simulink model "different_estimation_methods"  (R2023a)
settings: Solver=FixedStepAuto  StartTime=start_time  StopTime=stop_time  FixedStep=sample_time  RelTol=1e-3
values from neighbouring files (symbols this model uses):
  a = -0.8    [example12.m]    (also in example14.m; example15.m; example16.m)
  b = 0.5    [example12.m]    (also in example14.m; example15.m; example16.m)
  c = -0.5    [example12.m]    (also in example14.m = 0; example15.m = 0; example16.m = 0)
  e_mean = 0    [example15.m]    (also in example16.m)
  e_seed = 2    [example15.m]    (also in example16.m)
  e_var = e_std^2    (= 0.25)    [example15.m]    (also in example16.m)
  lambda = Lambda(i)    [example15.m]    (also in example16.m = 0.2)
  n_a = 1    [example15.m]    (also in example16.m)
  n_b = 1    [example15.m]    (also in example16.m)
  n_c = 0    [example15.m]    (also in example16.m = 1)
  P0 = 100 * eye(3)    [example12.m]    (also in example14.m = 0.01 * eye(2); example15.m = 100; example16.m = 0.01)
  sample_time = 1    [example12.m]    (also in example14.m; example15.m; example16.m)
  stop_time = 1000    [example12.m]    (also in example14.m = 20000; example15.m; example16.m = 5000)
  theta0 = zeros(3,1)    [example12.m]    (also in example14.m = Theta(:,i); example15.m = zeros(n_phi, 1); example16.m = zeros(n_phi, 1))
libraries: simulink x5
Description:
  | Three different projection algorithms compared with the RLS method.
  | Algorihtms:
  | 1) Least mean squares (LMS)
  | 2) Projection algorithm (PA)
  | 3) Stochastic approximation (SA)
settings Model: Creator=Beigi  LastModifiedBy=Mmoha

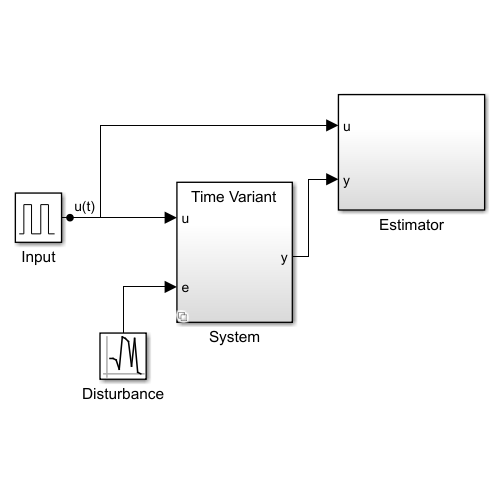
[thumbnail: Simulink's stored preview of the top-level diagram]
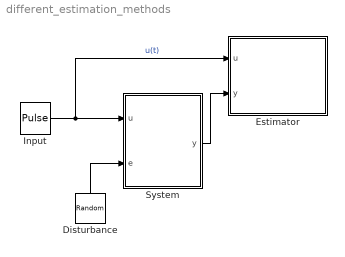
== system different_estimation_methods ==
  Disturbance : RandomNumber  Mean=e_mean  Variance=e_var  Seed=e_seed  SampleTime=sample_time
  Estimator : Subsystem
  Input : DiscretePulseGenerator  PulseType=Time based  Period=100  PulseWidth=50
  System : Subsystem  Variant=on  VariantControl=Choice
  wires:
  Input/1 -> Estimator/1(u), System/1(u)  "u(t)"
  Disturbance/1 -> System/2(e)
  System/1(y) -> Estimator/2(y)

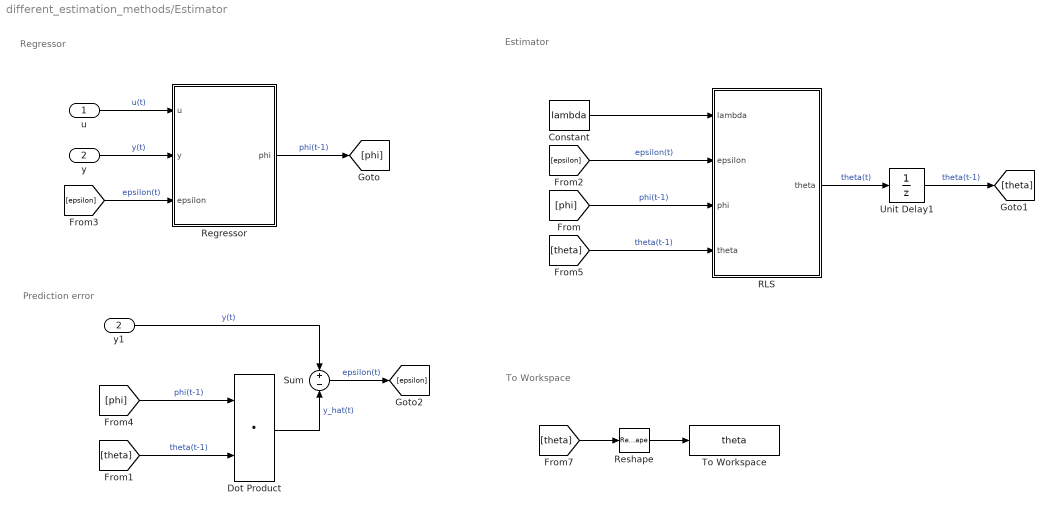
== system different_estimation_methods/Estimator ==
  note: To Workspace
  note: Estimator
  note: Prediction error
  note: Regressor
  u : Inport
  y : Inport  Port=2
  Constant : Constant  Value=lambda
  Dot Product : DotProduct  OutDataTypeStr=Inherit: Inherit via internal rule
  RLS : Subsystem  Variant=on  VariantControl=Choice
  Regressor : Subsystem  Variant=on  VariantControl=Choice
  Reshape : Reshape
  Sum : Sum  Inputs=+|-
  To Workspace : ToWorkspace  VariableName=theta  SaveFormat=Timeseries  SampleTime=-1
  Unit Delay1 : UnitDelay  InitialCondition=theta0  SampleTime=sample_time  HasFrameUpgradeWarning=on
  y1 : InportShadow  Port=2
  wires:
  Dot Product/1 -> Sum/2  "y_hat(t)"
  y1/1 -> Sum/1  "y(t)"
  Unit Delay1/1 -> [theta]  "theta(t-1)"
  Regressor/1(phi) -> [phi]  "phi(t-1)"
  [phi] -> Dot Product/1  "phi(t-1)"
  [theta] -> Dot Product/2  "theta(t-1)"
  Sum/1 -> [epsilon]  "epsilon(t)"
  [theta] -> Reshape/1
  u/1 -> Regressor/1(u)  "u(t)"
  y/1 -> Regressor/2(y)  "y(t)"
  [epsilon] -> Regressor/3(epsilon)  "epsilon(t)"
  Reshape/1 -> To Workspace/1
  Constant/1 -> RLS/1(lambda)
  [epsilon] -> RLS/2(epsilon)  "epsilon(t)"
  [phi] -> RLS/3(phi)  "phi(t-1)"
  [theta] -> RLS/4("theta ")  "theta(t-1)"
  RLS/1(theta) -> Unit Delay1/1  "theta(t)"

== system different_estimation_methods/System ==
  u : Inport
  e : Inport  Port=2
  Time Invariant : Subsystem  VariantControl=(default)
  Time Variant : Subsystem  VariantControl=time_variant == 1
  y : Outport

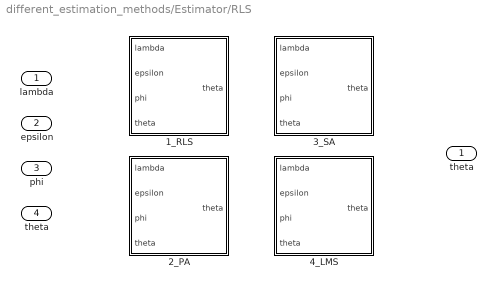
== system different_estimation_methods/Estimator/RLS ==
  lambda : Inport
  epsilon : Inport  Port=2
  phi : Inport  Port=3
  "theta " : Inport  Port=4
  1_RLS : Subsystem  VariantControl=(default)
  2_PA : Subsystem  VariantControl=estimation_method == 2
  3_SA : Subsystem  VariantControl=estimation_method == 3
  4_LMS : Subsystem  VariantControl=estimation_method == 4
  theta : Outport

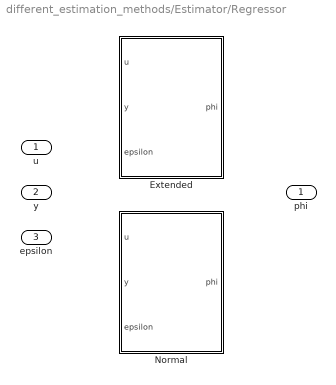
== system different_estimation_methods/Estimator/Regressor ==
  u : Inport
  y : Inport  Port=2
  epsilon : Inport  Port=3
  Extended : Subsystem  VariantControl=n_c > 0
  Normal : Subsystem  VariantControl=(default)
  phi : Outport

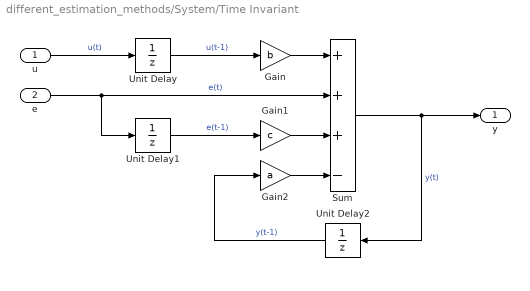
== system different_estimation_methods/System/Time Invariant ==
  u : Inport
  e : Inport  Port=2
  Gain : Gain  Gain=b
  Gain1 : Gain  Gain=c
  Gain2 : Gain  Gain=a
  Sum : Sum  Inputs=+++-
  Unit Delay : UnitDelay  SampleTime=sample_time  HasFrameUpgradeWarning=on
  Unit Delay1 : UnitDelay  SampleTime=sample_time  HasFrameUpgradeWarning=on
  Unit Delay2 : UnitDelay  SampleTime=sample_time  HasFrameUpgradeWarning=on
  y : Outport
  wires:
  Unit Delay/1 -> Gain/1  "u(t-1)"
  Gain/1 -> Sum/1
  Sum/1 -> y/1, Unit Delay2/1  "y(t)"
  e/1 -> Unit Delay1/1, Sum/2  "e(t)"
  Gain1/1 -> Sum/3
  Gain2/1 -> Sum/4
  u/1 -> Unit Delay/1  "u(t)"
  Unit Delay1/1 -> Gain1/1  "e(t-1)"
  Unit Delay2/1 -> Gain2/1  "y(t-1)"

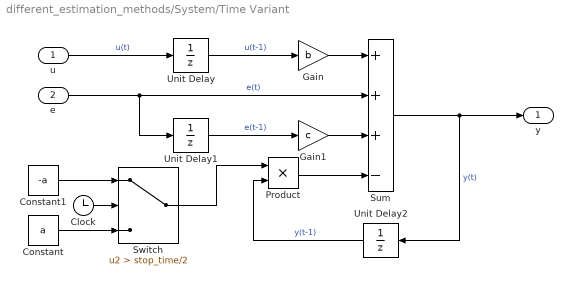
== system different_estimation_methods/System/Time Variant ==
  u : Inport
  e : Inport  Port=2
  Clock : Clock
  Constant : Constant  Value=a
  Constant1 : Constant  Value=-a
  Gain : Gain  Gain=b
  Gain1 : Gain  Gain=c
  Product : Product
  Sum : Sum  Inputs=+++-
  Switch : Switch  Criteria=u2 > Threshold  Threshold=stop_time/2  SaturateOnIntegerOverflow=off  InputSameDT=off
  Unit Delay : UnitDelay  SampleTime=sample_time  HasFrameUpgradeWarning=on
  Unit Delay1 : UnitDelay  SampleTime=sample_time  HasFrameUpgradeWarning=on
  Unit Delay2 : UnitDelay  SampleTime=sample_time  HasFrameUpgradeWarning=on
  y : Outport
  wires:
  Product/1 -> Sum/4
  Unit Delay2/1 -> Product/2  "y(t-1)"
  Unit Delay1/1 -> Gain1/1  "e(t-1)"
  Gain/1 -> Sum/1
  Gain1/1 -> Sum/3
  Sum/1 -> y/1, Unit Delay2/1  "y(t)"
  e/1 -> Unit Delay1/1, Sum/2  "e(t)"
  Unit Delay/1 -> Gain/1  "u(t-1)"
  u/1 -> Unit Delay/1  "u(t)"
  Clock/1 -> Switch/2
  Switch/1 -> Product/1
  Constant/1 -> Switch/3
  Constant1/1 -> Switch/1

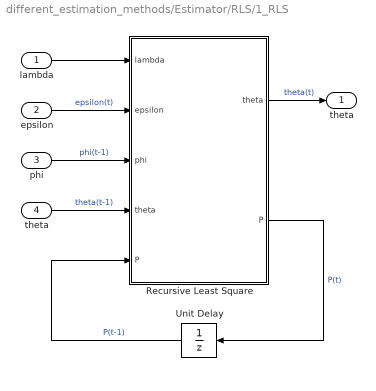
== system different_estimation_methods/Estimator/RLS/1_RLS ==
  lambda : Inport
  epsilon : Inport  Port=2
  phi : Inport  Port=3
  "theta " : Inport  Port=4
  Recursive Least Square : MATLAB Function  TreatAsAtomicUnit=on  VariantControl=(default)
  Unit Delay : UnitDelay  InitialCondition=P0  SampleTime=sample_time  HasFrameUpgradeWarning=on
  theta : Outport
  wires:
  Recursive Least Square/1(theta) -> theta/1  "theta(t)"
  "theta "/1 -> Recursive Least Square/4("theta ")  "theta(t-1)"
  Unit Delay/1 -> Recursive Least Square/5("P ")  "P(t-1)"
  lambda/1 -> Recursive Least Square/1(lambda)
  Recursive Least Square/2(P) -> Unit Delay/1  "P(t)"
  epsilon/1 -> Recursive Least Square/2(epsilon)  "epsilon(t)"
  phi/1 -> Recursive Least Square/3(phi)  "phi(t-1)"

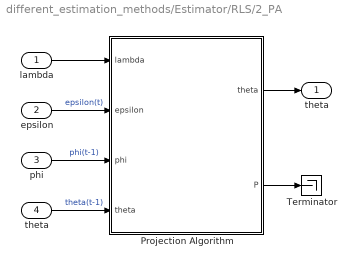
== system different_estimation_methods/Estimator/RLS/2_PA ==
  lambda : Inport
  epsilon : Inport  Port=2
  phi : Inport  Port=3
  "theta " : Inport  Port=4
  Projection Algorithm : MATLAB Function  TreatAsAtomicUnit=on  VariantControl=(default)
  Terminator : Terminator
  theta : Outport
  wires:
  lambda/1 -> Projection Algorithm/1(lambda)
  Projection Algorithm/2(P) -> Terminator/1
  Projection Algorithm/1(theta) -> theta/1
  "theta "/1 -> Projection Algorithm/4("theta ")  "theta(t-1)"
  phi/1 -> Projection Algorithm/3(phi)  "phi(t-1)"
  epsilon/1 -> Projection Algorithm/2(epsilon)  "epsilon(t)"

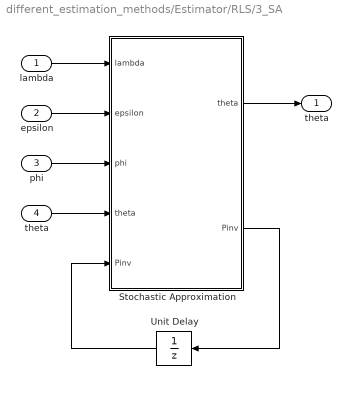
== system different_estimation_methods/Estimator/RLS/3_SA ==
  lambda : Inport
  epsilon : Inport  Port=2
  phi : Inport  Port=3
  "theta " : Inport  Port=4
  Stochastic Approximation : MATLAB Function  TreatAsAtomicUnit=on  VariantControl=(default)
  Unit Delay : UnitDelay  InitialCondition=P0  SampleTime=sample_time  HasFrameUpgradeWarning=on
  theta : Outport
  wires:
  epsilon/1 -> Stochastic Approximation/2(epsilon)
  lambda/1 -> Stochastic Approximation/1(lambda)
  phi/1 -> Stochastic Approximation/3(phi)
  "theta "/1 -> Stochastic Approximation/4("theta ")
  Stochastic Approximation/1(theta) -> theta/1
  Stochastic Approximation/2(Pinv) -> Unit Delay/1
  Unit Delay/1 -> Stochastic Approximation/5("Pinv ")

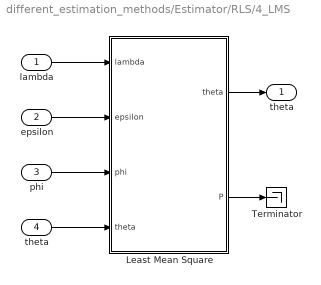
== system different_estimation_methods/Estimator/RLS/4_LMS ==
  lambda : Inport
  epsilon : Inport  Port=2
  phi : Inport  Port=3
  "theta " : Inport  Port=4
  Least Mean Square : MATLAB Function  TreatAsAtomicUnit=on  VariantControl=(default)
  Terminator : Terminator
  theta : Outport
  wires:
  "theta "/1 -> Least Mean Square/4("theta ")
  phi/1 -> Least Mean Square/3(phi)
  epsilon/1 -> Least Mean Square/2(epsilon)
  lambda/1 -> Least Mean Square/1(lambda)
  Least Mean Square/2(P) -> Terminator/1
  Least Mean Square/1(theta) -> theta/1

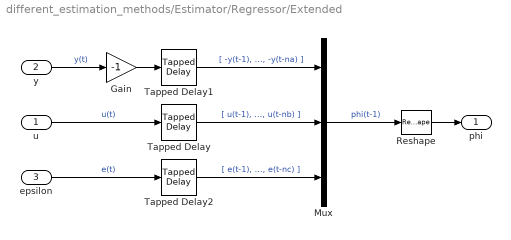
== system different_estimation_methods/Estimator/Regressor/Extended ==
  u : Inport
  y : Inport  Port=2
  epsilon : Inport  Port=3
  Gain : Gain  Gain=-1
  Mux : Mux  Inputs=3
  Reshape : Reshape  OutputDimensionality=Column vector (2-D)
  Tapped Delay : simulink/Discrete/Tapped Delay  vinit=0.0  samptime=sample_time  NumDelays=n_b  DelayOrder=Newest  includeCurrent=off
  Tapped Delay1 : simulink/Discrete/Tapped Delay  vinit=0.0  samptime=sample_time  NumDelays=n_a  DelayOrder=Newest  includeCurrent=off
  Tapped Delay2 : simulink/Discrete/Tapped Delay  vinit=0.0  samptime=sample_time  NumDelays=n_c  DelayOrder=Newest  includeCurrent=off
  phi : Outport
  wires:
  Reshape/1 -> phi/1
  u/1 -> Tapped Delay/1  "u(t)"
  y/1 -> Gain/1  "y(t)"
  epsilon/1 -> Tapped Delay2/1  "e(t)"
  Tapped Delay1/1 -> Mux/1  "[ -y(t-1), ..., -y(t-na) ]"
  Tapped Delay/1 -> Mux/2  "[ u(t-1), ..., u(t-nb) ]"
  Gain/1 -> Tapped Delay1/1
  Tapped Delay2/1 -> Mux/3  "[ e(t-1), ..., e(t-nc) ]"
  Mux/1 -> Reshape/1  "phi(t-1)"

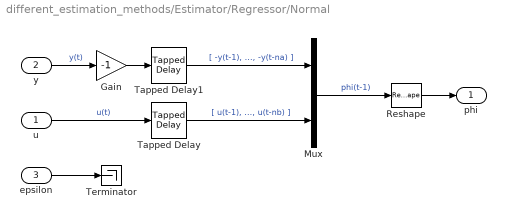
== system different_estimation_methods/Estimator/Regressor/Normal ==
  u : Inport
  y : Inport  Port=2
  epsilon : Inport  Port=3
  Gain : Gain  Gain=-1
  Mux : Mux  Inputs=2
  Reshape : Reshape  OutputDimensionality=Column vector (2-D)
  Tapped Delay : simulink/Discrete/Tapped Delay  vinit=0.0  samptime=sample_time  NumDelays=n_b  DelayOrder=Newest  includeCurrent=off
  Tapped Delay1 : simulink/Discrete/Tapped Delay  vinit=0.0  samptime=sample_time  NumDelays=n_a  DelayOrder=Newest  includeCurrent=off
  Terminator : Terminator
  phi : Outport
  wires:
  Mux/1 -> Reshape/1  "phi(t-1)"
  Gain/1 -> Tapped Delay1/1
  Tapped Delay/1 -> Mux/2  "[ u(t-1), ..., u(t-nb) ]"
  Tapped Delay1/1 -> Mux/1  "[ -y(t-1), ..., -y(t-na) ]"
  y/1 -> Gain/1  "y(t)"
  u/1 -> Tapped Delay/1  "u(t)"
  Reshape/1 -> phi/1
  epsilon/1 -> Terminator/1

== matlab function different_estimation_methods/Estimator/RLS/1_RLS/Recursive Least Square ==
  data: lambda input size=1; theta output; epsilon input size=1; phi input size=[n_phi, 1]; theta input size=[n_phi, 1]; P input size=[n_phi, n_phi]; P output; n_phi parameter size=1
function [theta, P] = fcn(lambda, epsilon, phi, theta, P, n_phi)
K = P * phi / (lambda + phi'*P*phi);
P = (eye(n_phi) - K*phi') * P / lambda;
theta = theta + P * phi * epsilon;

== matlab function different_estimation_methods/Estimator/RLS/2_PA/Projection Algorithm ==
  data: lambda input size=1; theta output; epsilon input size=1; phi input size=[n_phi, 1]; theta input size=[n_phi, 1]; P output; alpha parameter size=1
function [theta, P] = fcn(lambda, epsilon, phi, theta, alpha)

P = lambda / (alpha + phi' * phi);
theta = theta + P * phi * epsilon;

== matlab function different_estimation_methods/Estimator/RLS/3_SA/Stochastic Approximation ==
  data: lambda input size=1; theta output; epsilon input size=1; phi input size=[n_phi, 1]; theta input size=[n_phi, 1]; Pinv input size=1; Pinv output
function [theta, Pinv] = fcn(lambda, epsilon, phi, theta, Pinv)
Pinv = Pinv + phi'*phi;
P = lambda / Pinv;
theta = theta + P * phi * epsilon;

== matlab function different_estimation_methods/Estimator/RLS/4_LMS/Least Mean Square ==
  data: lambda input size=1; theta output; epsilon input size=1; phi input size=[n_phi, 1]; theta input size=[n_phi, 1]; P output
function [theta, P] = fcn(lambda, epsilon, phi, theta)

P = lambda;
theta = theta + P * phi * epsilon;
